simulink model "rotation_test"  (R2016b)
settings: Solver=VariableStepAuto  StartTime=0.0  StopTime=1000  RelTol=1e-3
libraries: dynamics_lib x2, rotation_visualization x1
settings Model: Creator=Sean  LastModifiedBy=Sean

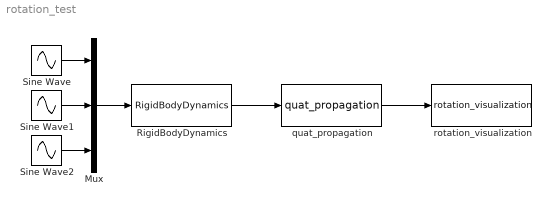
== system rotation_test ==
  Mux : Mux  Inputs=3
  RigidBodyDynamics : dynamics_lib/Dynamics/RigidBodyDynamics
  Sine Wave : Sin  Amplitude=2e-4  SampleTime=0
  Sine Wave1 : Sin  Amplitude=2e-4  Phase=pi/3  SampleTime=0
  Sine Wave2 : Sin  Amplitude=2e-4  Phase=2*pi/3  SampleTime=0
  quat_propagation : dynamics_lib/Dynamics/quat_propagation
  rotation_visualization : rotation_visualization/rotation_visualization
  wires:
  Mux/1 -> RigidBodyDynamics/1
  Sine Wave1/1 -> Mux/2
  Sine Wave/1 -> Mux/1
  Sine Wave2/1 -> Mux/3
  RigidBodyDynamics/1 -> quat_propagation/1
  quat_propagation/1 -> rotation_visualization/1
